simulink model "DCM_17_Series_Field_2_With_2_Motors_Discharge"  (R2019b)
settings: Solver=VariableStepAuto  StartTime=0.0  StopTime=200  RelTol=1e-3
model workspace (MAT data in the model file):
  Laf = 0.008
  Laf_2 = 0.00844
  Rarm = 0.0096
  angular_vel = 163.55
  angular_vel_1 = 175.405
  angular_vel_10 = 168.703
  angular_vel_11 = 168.598
  angular_vel_12 = 167.865
  angular_vel_13 = 167.132
  angular_vel_14 = 166.923
  angular_vel_15 = 165.666
  angular_vel_16 = 164.41
  angular_vel_2 = 173.625
  angular_vel_3 = 172.787
  angular_vel_4 = 170.902
  angular_vel_5 = 170.902
  angular_vel_6 = 169.96
  angular_vel_7 = 169.855
  angular_vel_8 = 169.122
libraries: powerlib x14
settings Model: OrderedModelArguments=off  Creator=Sy2  LastModifiedBy=Sy2
settings SolverCC: ZeroCrossAlgorithm=Adaptive
settings DebuggingCC: IgnoredZcDiagnostic=none

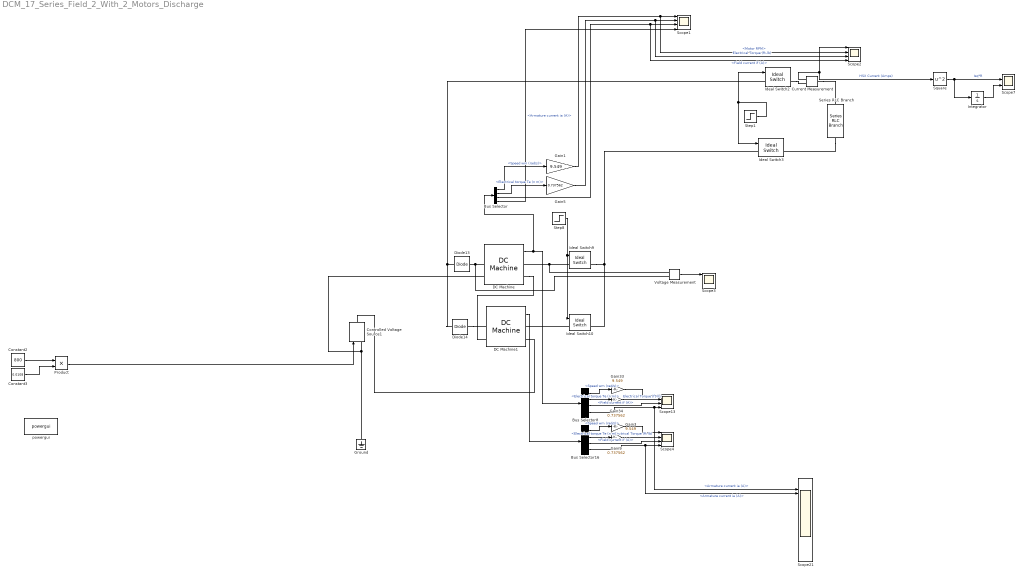
== system DCM_17_Series_Field_2_With_2_Motors_Discharge ==
  Bus Selector : BusSelector  OutputSignals=Speed wm (rad/s),Electrical torque Te (n m),Field current if (A),Armature current ia (A)
  Bus Selector16 : BusSelector  OutputSignals=Speed wm (rad/s),Electrical torque Te (n m),Field current if (A),Armature current ia (A)
  Bus Selector8 : BusSelector  OutputSignals=Speed wm (rad/s),Electrical torque Te (n m),Field current if (A),Armature current ia (A)
  Constant2 : Constant  Value=800
  Constant3 : Constant  Value=0.0108
  Controlled Voltage Source1 : powerlib/Electrical Sources/Controlled Voltage Source  Initialize=on  Source_Type=DC  Amplitude=0  Phase=0  Frequency=0  Measurements=Voltage
      settings: SourceProductName=Simscape Electrical
  Current Measurement : powerlib/Measurements/Current Measurement  PhasorSimulation=off  OutputType=Complex  PSBequivalent=0
      settings: SourceProductName=Simscape Electrical
  DC Machine : powerlib/Machines/DC Machine  PresetModel=No  MechanicalLoad=Torque TL  FieldType=Wound  ShowDetailedParameters=on  MeasurementBus=off  RLa="[Rarm  0.002]"  RLf=[0.0054 0.0125]  Laf=Laf  MachineConstant=Torque constant (N.m/A)  Ke=1.8  Kt=1.8  J=137  Bm=0  Tf=0  w0=angular_vel  Ifinit=0  TsPowergui=0  TsBlock=-1
      settings: SourceProductName=Simscape Electrical
  DC Machine1 : powerlib/Machines/DC Machine  PresetModel=No  MechanicalLoad=Torque TL  FieldType=Wound  ShowDetailedParameters=on  MeasurementBus=off  RLa="[Rarm  0.002]"  RLf=[0.0054 0.0125]  Laf=Laf  MachineConstant=Torque constant (N.m/A)  Ke=1.8  Kt=1.8  J=137  Bm=0  Tf=0  w0=angular_vel  Ifinit=0  TsPowergui=0  TsBlock=-1
      settings: SourceProductName=Simscape Electrical
  Diode13 : powerlib/Power Electronics/Diode  Ron=0.001  Lon=0  Vf=0.8  IC=0  UseSnubber=0  Rs=500000  Cs=250e-9  Measurements=off
      settings: SourceProductName=Simscape Electrical
  Diode14 : powerlib/Power Electronics/Diode  Ron=0.001  Lon=0  Vf=0.8  IC=0  UseSnubber=0  Rs=500000  Cs=250e-9  Measurements=off
      settings: SourceProductName=Simscape Electrical
  Gain1 : Gain  Gain=9.549
  Gain3 : Gain  Gain=9.549
  Gain33 : Gain  Gain=9.549
  Gain34 : Gain  Gain=0.737562
  Gain5 : Gain  Gain=0.737562
  Gain9 : Gain  Gain=0.737562
  Ground : powerlib/Elements/Ground  LConnTagsString=a
      settings: SourceProductName=Simscape Electrical
  Ideal Switch{2..3,9..10} (4 alike) : powerlib/Power Electronics/Ideal Switch  Ron=0  Lon=0  IC=0  Rs=inf  Cs=0  Measurements=on
      settings: SourceProductName=Simscape Electrical
  Integrator : Integrator  ZeroCross=off
  Product : Product
  Scope{1..4,13} (5 alike) : Scope  NumInputPorts=4
  Scope21 : Scope  NumInputPorts=16
  Scope7 : Scope  NumInputPorts=2
  Series RLC Branch : powerlib/Elements/Series RLC Branch  LConnTagsString=__new0  RConnTagsString=__new0  BranchType=RL  Resistance=0.1  Inductance=0.02  SetiL0=off  InitialCurrent=0  Capacitance=1e-6  Setx0=off  InitialVoltage=0  Measurements=None
      settings: SourceProductName=Simscape Electrical
  Square : Math  Operator=square  RndMeth=Zero  SaturateOnIntegerOverflow=on
  Step1 : Step  Time=14  SampleTime=0  VectorParams1D=off
  Step8 : Step  Time=14  SampleTime=0  VectorParams1D=off  ZeroCross=off
  Voltage Measurement : powerlib/Measurements/Voltage Measurement  PhasorSimulation=off  OutputType=Complex  PSBequivalent=0
      settings: SourceProductName=Simscape Electrical
  powergui : powerlib/powergui  Priority=1  SimulationMode=Continuous  SampleTime=50e-6  frequency=60  Iterations=50  frequencyindice=0  Pbase=100e6  ErrMax=1e-4  UnitsV=kV  UnitsW=MW  buscounter=0  FunctionMessages=off  echomessages=off  EnableUseOfTLC=off  CurrentSourceSwitches=off  DisableSnubberDevices=off  DisableRonSwitches=off  DisableVfSwitches=off  DisplayEquations=off  AutomaticDiscreteSolvers=off  SolverType=Tustin/Backward Euler (TBE)  Interpol=off  ExternalGateDelay=off  methode=off  Ts=100  x0status=blocks  SPID=on  SwTol=0  HookPort=off  NonlinearTolerance=1e-4  nMaxIteration=100  ContinueOnMaxIteration=off  RestoreLinks=warning  ResistiveCurrentMeasurement=off  Frange=[0:2:500]  Ylog=off  Xlog=on  ShowGrid=off  save=off  variable=ZData  structure=0  ZoomFFT=off  StartTime=0.0  cycles=1  DisplayStyle=1  fundamental=60  FreqAxis=off  MaxFrequency=1000  frequencyindicesteady=1  RmsSteady=1  display=off
      settings: SourceProductName=Simscape Electrical
  wires:
  Bus Selector/1 -> Gain1/1  "<Speed wm (rad/s)>"
  Bus Selector/3 -> Scope2/4, Scope1/3  "<Field current if (A)>"
  Bus Selector/4 -> Scope1/4  "<Armature current ia (A)>"
  Gain1/1 -> Scope1/1, Scope2/2  "<Motor RPM>"
  Step1/1 -> Ideal Switch2/1, Ideal Switch3/1
  Current Measurement/1 -> Square/1, Scope2/1  "HSX Current (Amps)"
  Constant2/1 -> Product/1
  Bus Selector/2 -> Gain5/1  "<Electrical torque Te (n m)>"
  Gain5/1 -> Scope2/3, Scope1/2  "Electrical Torque (ft-lb)"
  Square/1 -> Scope7/1, Integrator/1  "Isq*R"
  Integrator/1 -> Scope7/2
  Product/1 -> Controlled Voltage Source1/1
  Constant3/1 -> Product/2
  Bus Selector8/3 -> Scope13/3  "<Field current if (A)>"
  Bus Selector8/2 -> Gain34/1  "<Electrical torque Te (n m)>"
  Gain34/1 -> Scope13/2  "Electrical Torque (ft-lb)"
  Bus Selector8/1 -> Gain33/1  "<Speed wm (rad/s)>"
  Gain33/1 -> Scope13/1
  Bus Selector8/4 -> Scope21/1, Scope13/4  "<Armature current ia (A)>"
  DC Machine/1 -> Bus Selector8/1, Bus Selector/1
  DC Machine1/1 -> Bus Selector16/1
  Gain3/1 -> Scope4/1
  Gain9/1 -> Scope4/2  "Electrical Torque (ft-lb)"
  Bus Selector16/1 -> Gain3/1  "<Speed wm (rad/s)>"
  Bus Selector16/3 -> Scope4/3  "<Field current if (A)>"
  Bus Selector16/2 -> Gain9/1  "<Electrical torque Te (n m)>"
  Bus Selector16/4 -> Scope21/2, Scope4/4  "<Armature current ia (A)>"
  Step8/1 -> Ideal Switch10/1, Ideal Switch9/1
  Voltage Measurement/1 -> Scope3/1
  connections:
  Ideal Switch9/RConn1 -- Ideal Switch10/RConn1 -- Ideal Switch3/LConn1
  Series RLC Branch/RConn1 -- Ideal Switch3/RConn1
  Ideal Switch2/LConn1 -- Diode14/LConn1 -- Diode13/LConn1
  DC Machine/RConn2 -- DC Machine1/LConn2
  Ideal Switch9/LConn1 -- Voltage Measurement/LConn1 -- DC Machine/RConn1
  Ideal Switch10/LConn1 -- DC Machine1/RConn1
  Diode14/RConn1 -- DC Machine1/LConn1
  Diode13/RConn1 -- Voltage Measurement/LConn2 -- DC Machine/LConn1
  Ground/LConn1 -- DC Machine/LConn2 -- Controlled Voltage Source1/LConn1
  Ideal Switch2/RConn1 -- Current Measurement/RConn1
  Current Measurement/LConn1 -- Series RLC Branch/LConn1
  Controlled Voltage Source1/RConn1 -- DC Machine1/RConn2
